simulink model "simsimulink"  (R2024a)
settings: Solver=ode8  StartTime=0.0  StopTime=10  FixedStep=0.000001  RelTol=1e-3
values from neighbouring files (symbols this model uses):
  am = 1/(Rlnom*C)    (= 53.1914893617)    [params.m]
  bm = 1    [params.m]
  C = 470e-6    (= 0.00047)    [params.m]
  E = 100    [params.m]
  k1 = 5000000    [params.m]
  k2 = 400000    [params.m]
  k3 = 700000    [params.m]
  kappa = 320    [params.m]
  L = 0.5e-3    (= 0.0005)    [params.m]
  omega = 100*pi    (= 314.159265359)    [params.m]
  Qas = bm    (= 1)    [params.m]
  R = 0.1    [params.m]
  Rlnom = 40    [params.m]
  Thetaas = 0    [params.m]
  vod = 200    [params.m]
  w = 100    [params.m]
libraries: spsIGBTDiodeLib x6, spsVoltageMeasurementLib x5, spsCurrentMeasurementLib x4, spsSeriesRLCBranchLib x4, spsACVoltageSourceLib x3, simulink x3, eeTransforms x2, spsControlledVoltageSourceLib x1, spsGroundLib x1, spsSVPWMGenerator2LevelLib x1, spsVariableResistorLib x1, spspowerguiLib x1
settings Model: Creator=rodol  LastModifiedBy=rodol

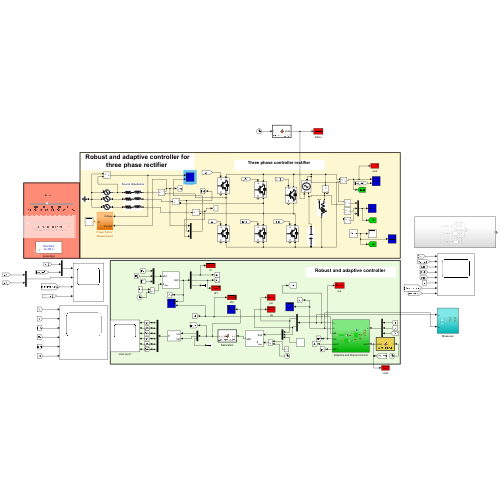
[thumbnail: Simulink's stored preview of the top-level diagram]
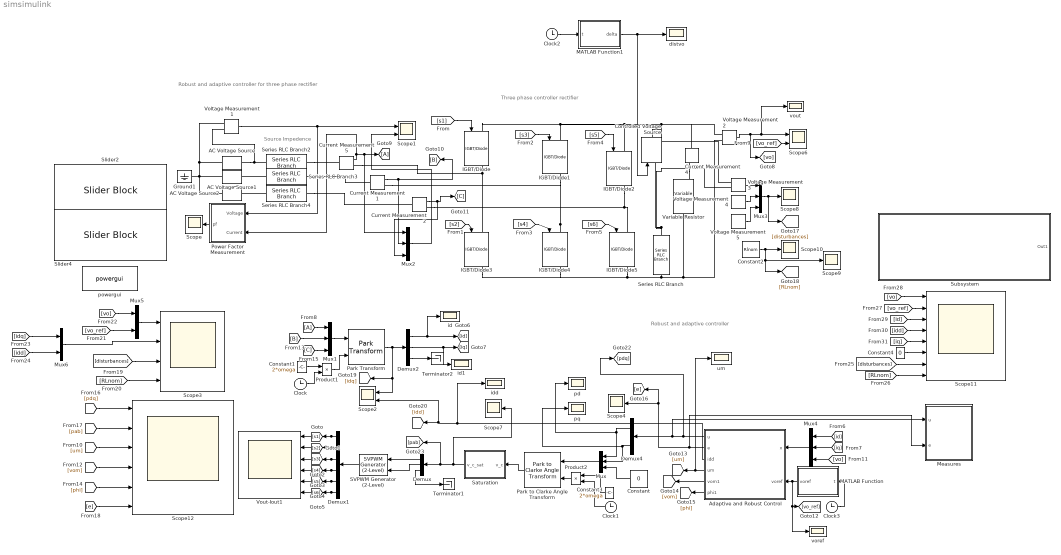
== system simsimulink ==
  note: Robust and adaptive controller
  note: Three phase controller rectifier
  note: Source Impedence
  note: Robust and adaptive controller for three phase rectifier
  " pq" : Scope
  AC Voltage Source : spsACVoltageSourceLib/AC Voltage Source  Amplitude=E  Phase=0  Frequency=w  SampleTime=0  Measurements=None  BusType=swing  Pref=10e3  Qref=0  Qmin=-inf  Qmax=+inf
  AC Voltage Source1 : spsACVoltageSourceLib/AC Voltage Source  Amplitude=E  Phase=240  Frequency=w  SampleTime=0  Measurements=None  BusType=swing  Pref=10e3  Qref=0  Qmin=-inf  Qmax=+inf
  AC Voltage Source2 : spsACVoltageSourceLib/AC Voltage Source  Amplitude=E  Phase=120  Frequency=w  SampleTime=0  Measurements=None  BusType=swing  Pref=10e3  Qref=0  Qmin=-inf  Qmax=+inf
  Adaptive and Robust Control : Subsystem
  Clock{,1..3} (4 alike) : Clock
  Constant : Constant  Value=0
  Constant1 : Constant  Value=2*omega
  Constant2 : Constant  Value=Rlnom
  Constant3 : Constant  Value=2*omega
  Constant4 : Constant  Value=0
  Controlled Voltage Source : spsControlledVoltageSourceLib/Controlled Voltage Source  Initialize=on  Source_Type=DC  Amplitude=0  Phase=0  Frequency=0  Measurements=None
  Current Measurement{1..2,4..5} (4 alike) : spsCurrentMeasurementLib/Current Measurement  PhasorSimulation=off  OutputType=Magnitude  PSBequivalent=0
  Demux : Demux  Outputs=3
  Demux1 : Demux  Outputs=6
  Demux2 : Demux  Outputs=3
  Demux4 : Demux  Outputs=2
  From8 : From
  Goto9 : Goto
  Ground1 : spsGroundLib/Ground  LConnTagsString=a
  IGBT/Diode{,1..5} (6 alike) : spsIGBTDiodeLib/IGBT//Diode  Ron=1e-3  Rs=1e5  Cs=inf  Measurements=on
  MATLAB Function : MATLAB Function  TreatAsAtomicUnit=on
  MATLAB Function1 : MATLAB Function  TreatAsAtomicUnit=on
  Measures : Subsystem
  Mux{,1..4} (5 alike) : Mux  Inputs=3
  Mux5 : Mux  Inputs=2
  Mux6 : Mux  Inputs=2
  Park Transform : eeTransforms/Park Transform  AxisAlignment=D-axis  PowerInvariant=off
  Park to Clarke Angle Transform : eeTransforms/Park to Clarke Angle Transform  AxisAlignment=D-axis
  Power Factor Measurement : Subsystem
  Product1 : Product
  Product2 : Product
  SVPWM Generator (2-Level) : spsSVPWMGenerator2LevelLib/SVPWM Generator (2-Level)  InputType=alpha-beta components  SwitchingPattern=Pattern #1  Fc=80000  ParUref=[0.8 -30 50]  Ts=0.000001
  Saturation : MATLAB Function  TreatAsAtomicUnit=on
  Scope{,4,7..10} (6 alike) : Scope
  Scope1 : Scope  NumInputPorts=2
  Scope11 : Scope  NumInputPorts=8
  Scope12 : Scope  NumInputPorts=6
  Scope2 : Scope  NumInputPorts=2
  Scope3 : Scope  NumInputPorts=4
  Scope6 : Scope  NumInputPorts=2
  Series RLC Branch : spsSeriesRLCBranchLib/Series RLC Branch  LConnTagsString=__new0  RConnTagsString=__new0  BranchType=C  Resistance=5  Inductance=1e-3  SetiL0=off  InitialCurrent=0  Capacitance=C  Setx0=off  InitialVoltage=0  Measurements=None
  Series RLC Branch2 : spsSeriesRLCBranchLib/Series RLC Branch  LConnTagsString=__new0  RConnTagsString=__new0  BranchType=RL  Resistance=R  Inductance=L  SetiL0=off  InitialCurrent=0  Capacitance=200e-6  Setx0=off  InitialVoltage=0  Measurements=Branch voltage and current
  Series RLC Branch3 : spsSeriesRLCBranchLib/Series RLC Branch  LConnTagsString=__new0  RConnTagsString=__new0  BranchType=RL  Resistance=R  Inductance=L  SetiL0=off  InitialCurrent=0  Capacitance=200e-6  Setx0=off  InitialVoltage=0  Measurements=Branch voltage and current
  Series RLC Branch4 : spsSeriesRLCBranchLib/Series RLC Branch  LConnTagsString=__new0  RConnTagsString=__new0  BranchType=RL  Resistance=R  Inductance=L  SetiL0=off  InitialCurrent=0  Capacitance=200e-6  Setx0=off  InitialVoltage=0  Measurements=Branch voltage and current
  Slider2 : SliderBlock  ScaleMin=25
  Slider4 : SliderBlock  ScaleMax=5
  Subsystem : Subsystem
  Terminator1 : Terminator
  Terminator2 : Terminator
  Variable Resistor : spsVariableResistorLib/Variable Resistor  Rabsmin=Rlnom
  Voltage Measurement{1..5} (5 alike) : spsVoltageMeasurementLib/Voltage Measurement  PhasorSimulation=off  OutputType=Magnitude  PSBequivalent=0
  Vout-Iout1 : Scope  NumInputPorts=6
  distvo : Scope
  id : Scope
  id1 : Scope
  idd : Scope
  pd : Scope
  powergui : spspowerguiLib/powergui  Priority=1  SimulationMode=Discrete  SampleTime=1e-6  frequency=60  Iterations=50  frequencyindice=0  Pbase=100e6  ErrMax=1e-4  UnitsV=kV  UnitsW=MW  buscounter=0  FunctionMessages=off  echomessages=off  EnableUseOfTLC=off  CurrentSourceSwitches=off  DisableSnubberDevices=off  DisableRonSwitches=off  DisableVfSwitches=off  DisplayEquations=off  AutomaticDiscreteSolvers=off  SolverType=Tustin/Backward Euler (TBE)  Interpol=off  ExternalGateDelay=off  methode=off  Ts=0  x0status=blocks  SPID=off  SwTol=0  HookPort=off  NonlinearTolerance=0  nMaxIteration=15  ContinueOnMaxIteration=off  RestoreLinks=warning  ResistiveCurrentMeasurement=off  Frange=[0:2:500]  Ylog=off  Xlog=on  ShowGrid=off  save=off  variable=ZData  structure=0  ZoomFFT=on  StartTime=0.0  cycles=1  DisplayStyle=1  fundamental=60  FreqAxis=off  MaxFrequency=1000  frequencyindicesteady=1  RmsSteady=1  display=off
  um : Scope
  voref : Scope
  vout : Scope
  wires:
  Demux2/2 -> id1/1, [iq]
  Clock1/1 -> Product2/2
  Park Transform/1 -> [idq], Scope2/1, Demux2/1
  Current Measurement5/1 -> Mux2/1, Goto9/1, Power Factor Measurement/2(Current)
  [s5] -> IGBT/Diode2/1
  [s4] -> IGBT/Diode4/1
  Demux1/5 -> Vout-Iout1/5, [s5]
  Product1/1 -> Park Transform/2
  Constant1/1 -> Product1/1
  Demux1/1 -> Vout-Iout1/1, [s1]
  [s2] -> IGBT/Diode3/1
  Clock/1 -> Product1/2
  Demux2/1 -> id/1, [id]
  [s1] -> IGBT/Diode/1
  Power Factor Measurement/1(pf) -> Scope/1
  Demux2/3 -> Terminator2/1
  [s6] -> IGBT/Diode5/1
  Mux1/1 -> Park Transform/1
  Constant3/1 -> Product2/1
  Product2/1 -> Park to Clarke Angle Transform/2
  Demux1/3 -> Vout-Iout1/3, [s3]
  Demux1/4 -> Vout-Iout1/4, [s4]
  Demux1/2 -> Vout-Iout1/2, [s2]
  Demux/3 -> Terminator1/1
  Constant/1 -> Mux/3
  Voltage Measurement1/1 -> Scope1/1, Power Factor Measurement/1(Voltage)
  Demux1/6 -> Vout-Iout1/6, [s6]
  [s3] -> IGBT/Diode1/1
  Demux4/1 -> pd/1, Mux/1
  Demux4/2 -> " pq"/1, Mux/2
  Voltage Measurement2/1 -> [vo], vout/1, Scope6/1
  Mux4/1 -> Adaptive and Robust Control/1(x)
  Clock3/1 -> MATLAB Function/1(t)
  MATLAB Function/1(voref) -> voref/1, [vo_ref], Adaptive and Robust Control/2(voref)
  [vo] -> Mux4/3
  [id] -> Mux4/1
  [iq] -> Mux4/2
  From8/1 -> Mux1/1
  Current Measurement1/1 -> Mux2/2, [B]
  [B] -> Mux1/2
  Current Measurement2/1 -> Mux2/3, [C]
  [C] -> Mux1/3
  [vo_ref] -> Scope6/2
  Mux2/1 -> Scope1/2
  Mux/1 -> Park to Clarke Angle Transform/1
  Adaptive and Robust Control/3(idd) -> idd/1, [idd], Scope2/2
  Voltage Measurement3/1 -> Mux3/1
  Voltage Measurement4/1 -> Mux3/2
  Voltage Measurement5/1 -> Mux3/3
  Mux3/1 -> [disturbances], Scope8/1
  Constant2/1 -> Scope9/1, [RLnom], Scope10/1
  Adaptive and Robust Control/4(um) -> um/1, [um]
  Adaptive and Robust Control/6(phi1) -> [phi]
  Adaptive and Robust Control/5(vom1) -> [vom]
  [um] -> Scope12/3
  [vom] -> Scope12/4
  [phi] -> Scope12/5
  [pdq] -> Scope12/1
  [e] -> Scope12/6
  [vo] -> Mux5/1
  [vo_ref] -> Mux5/2
  [idq] -> Mux6/1
  [idd] -> Mux6/2
  Mux5/1 -> Scope3/1
  Mux6/1 -> Scope3/2
  [disturbances] -> Scope3/3
  [RLnom] -> Scope3/4
  [vo] -> Scope11/1
  [vo_ref] -> Scope11/2
  [id] -> Scope11/3
  [iq] -> Scope11/5
  [idd] -> Scope11/4
  Constant4/1 -> Scope11/6
  [disturbances] -> Scope11/7
  [RLnom] -> Scope11/8
  [pab] -> Scope12/2
  Clock2/1 -> MATLAB Function1/1(t)
  MATLAB Function1/1(delta) -> distvo/1, Controlled Voltage Source/1
  Adaptive and Robust Control/2(e) -> Measures/2(e), [e], Scope4/1
  Adaptive and Robust Control/1(u) -> [pdq], Measures/1(u), Demux4/1
  Demux/1 -> SVPWM Generator (2-Level)/1
  Demux/2 -> SVPWM Generator (2-Level)/2
  Park to Clarke Angle Transform/1 -> Saturation/1(v_c)
  SVPWM Generator (2-Level)/1 -> Demux1/1
  Saturation/1(v_c_sat) -> Scope7/1, [pab], Demux/1
  connections:
  IGBT/Diode1/LConn1 -- IGBT/Diode/LConn1 -- Voltage Measurement3/LConn1 -- Controlled Voltage Source/RConn1 -- Current Measurement4/LConn1 -- Voltage Measurement2/LConn1 -- IGBT/Diode2/LConn1
  IGBT/Diode2/RConn1 -- IGBT/Diode5/LConn1 -- Current Measurement2/RConn1
  Series RLC Branch3/RConn1 -- Current Measurement1/LConn1
  Series RLC Branch2/RConn1 -- Current Measurement5/LConn1
  Series RLC Branch4/RConn1 -- Current Measurement2/LConn1
  AC Voltage Source/RConn1 -- Voltage Measurement1/LConn1 -- AC Voltage Source2/RConn1 -- AC Voltage Source1/RConn1 -- Ground1/LConn1
  IGBT/Diode4/LConn1 -- IGBT/Diode1/RConn1 -- Current Measurement1/RConn1
  Current Measurement5/RConn1 -- IGBT/Diode/RConn1 -- IGBT/Diode3/LConn1
  Series RLC Branch3/LConn1 -- AC Voltage Source1/LConn1
  Voltage Measurement2/LConn2 -- IGBT/Diode4/RConn1 -- IGBT/Diode3/RConn1 -- IGBT/Diode5/RConn1 -- Series RLC Branch/RConn1 -- Variable Resistor/RConn1
  Series RLC Branch4/LConn1 -- AC Voltage Source2/LConn1
  AC Voltage Source/LConn1 -- Voltage Measurement1/LConn2 -- Series RLC Branch2/LConn1
  Current Measurement4/RConn1 -- Variable Resistor/LConn1
  Series RLC Branch/LConn1 -- Voltage Measurement3/LConn2 -- Controlled Voltage Source/LConn1

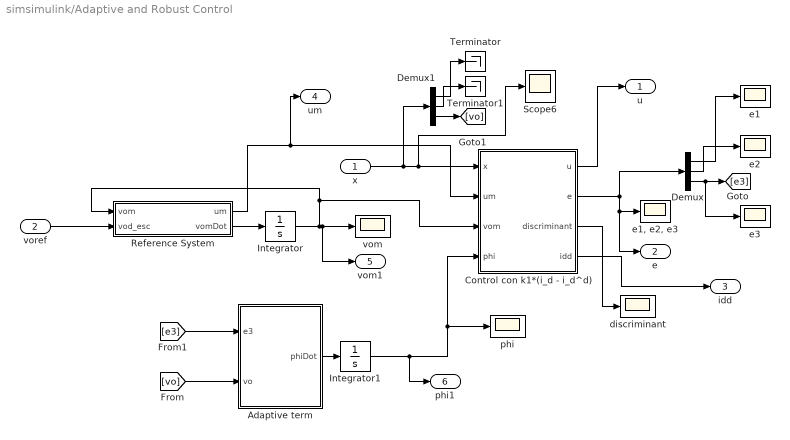
== system simsimulink/Adaptive and Robust Control ==
  x : Inport
  voref : Inport  Port=2
  " e1" : Scope
  " e2" : Scope
  " e3" : Scope
  Adaptive term : MATLAB Function  TreatAsAtomicUnit=on
  Control con k1*(i_d - i_d^d) : MATLAB Function  TreatAsAtomicUnit=on
  Demux : Demux  Outputs=3
  Demux1 : Demux  Outputs=3
  Integrator : Integrator
  Integrator1 : Integrator
  Reference System : MATLAB Function  TreatAsAtomicUnit=on
  Scope6 : Scope
  Terminator : Terminator
  Terminator1 : Terminator
  discriminant : Scope
  "e1, e2, e3" : Scope
  phi : Scope
  vom : Scope
  u : Outport
  e : Outport  Port=2
  idd : Outport  Port=3
  um : Outport  Port=4
  vom1 : Outport  Port=5
  phi1 : Outport  Port=6
  wires:
  x/1 -> Demux1/1, Scope6/1, Control con k1*(i_d - i_d^d)/1(x)
  Control con k1*(i_d - i_d^d)/3(discriminant) -> discriminant/1
  Control con k1*(i_d - i_d^d)/2(e) -> e/1, "e1, e2, e3"/1, Demux/1
  Control con k1*(i_d - i_d^d)/1(u) -> u/1
  Reference System/2(vomDot) -> Integrator/1
  Integrator/1 -> vom1/1, vom/1, Reference System/1(vom), Control con k1*(i_d - i_d^d)/3(vom)
  Adaptive term/1(phiDot) -> Integrator1/1
  Reference System/1(um) -> um/1, Control con k1*(i_d - i_d^d)/2(um)
  Integrator1/1 -> phi1/1, phi/1, Control con k1*(i_d - i_d^d)/4(phi)
  Demux/3 -> " e3"/1, [e3]
  Demux1/3 -> [vo]
  [e3] -> Adaptive term/1(e3)
  [vo] -> Adaptive term/2(vo)
  Demux1/1 -> Terminator/1
  Demux1/2 -> Terminator1/1
  voref/1 -> Reference System/2(vod_esc)
  Demux/1 -> " e1"/1
  Demux/2 -> " e2"/1
  Control con k1*(i_d - i_d^d)/4(idd) -> idd/1

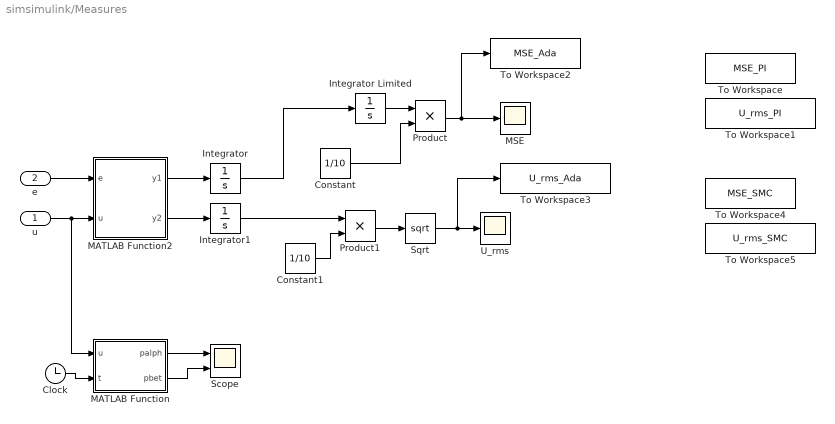
== system simsimulink/Measures ==
  u : Inport
  e : Inport  Port=2
  Clock : Clock
  Constant : Constant  Value=1/10
  Constant1 : Constant  Value=1/10
  Integrator : Integrator
  Integrator Limited : Integrator  UpperSaturationLimit=1  LowerSaturationLimit=0
  Integrator1 : Integrator
  MATLAB Function : MATLAB Function  TreatAsAtomicUnit=on
  MATLAB Function2 : MATLAB Function  TreatAsAtomicUnit=on
  MSE : Scope
  Product : Product
  Product1 : Product
  Scope : Scope  NumInputPorts=2
  Sqrt : Sqrt
  To Workspace : ToWorkspace  VariableName=MSE_PI  SaveFormat=Timeseries  SampleTime=-1
  To Workspace1 : ToWorkspace  VariableName=U_rms_PI  SaveFormat=Timeseries  SampleTime=-1
  To Workspace2 : ToWorkspace  VariableName=MSE_Ada  SaveFormat=Timeseries  SampleTime=-1
  To Workspace3 : ToWorkspace  VariableName=U_rms_Ada  SaveFormat=Timeseries  SampleTime=-1
  To Workspace4 : ToWorkspace  VariableName=MSE_SMC  SaveFormat=Timeseries  SampleTime=-1
  To Workspace5 : ToWorkspace  VariableName=U_rms_SMC  SaveFormat=Timeseries  SampleTime=-1
  U_rms : Scope
  wires:
  Integrator Limited/1 -> Product/1
  Constant/1 -> Product/2
  Product/1 -> To Workspace2/1, MSE/1
  Sqrt/1 -> To Workspace3/1, U_rms/1
  MATLAB Function2/2(y2) -> Integrator1/1
  Constant1/1 -> Product1/2
  Product1/1 -> Sqrt/1
  u/1 -> MATLAB Function/1(u), MATLAB Function2/2(u)
  e/1 -> MATLAB Function2/1(e)
  MATLAB Function2/1(y1) -> Integrator/1
  Integrator/1 -> Integrator Limited/1
  Integrator1/1 -> Product1/1
  Clock/1 -> MATLAB Function/2(t)
  MATLAB Function/1(palph) -> Scope/1
  MATLAB Function/2(pbet) -> Scope/2

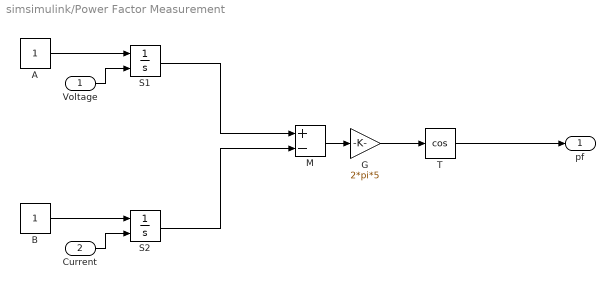
== system simsimulink/Power Factor Measurement ==
  Voltage : Inport
  Current : Inport  Port=2
  A : Constant
  B : Constant
  G : Gain  Gain=2*pi*5
  M : Sum  Inputs=+-
  S1 : Integrator  ExternalReset=falling
  S2 : Integrator  ExternalReset=falling
  T : Trigonometry  Operator=cos
  pf : Outport
  wires:
  A/1 -> S1/1
  B/1 -> S2/1
  S1/1 -> M/1
  S2/1 -> M/2
  Voltage/1 -> S1/2
  Current/1 -> S2/2
  M/1 -> G/1
  G/1 -> T/1
  T/1 -> pf/1

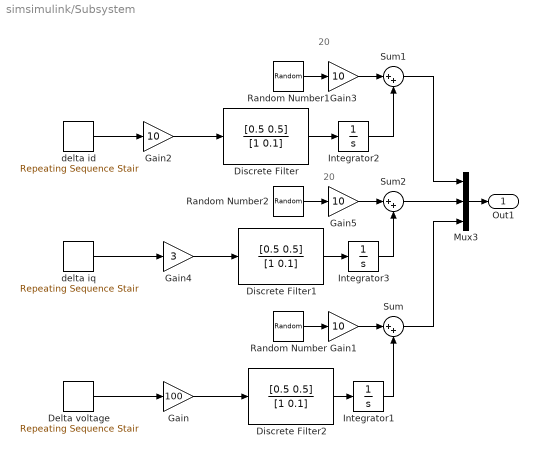
== system simsimulink/Subsystem ==
  note: 20
  note: 20
  Delta voltage : simulink/Sources/Repeating Sequence Stair  OutValues=[0 0 1 1 -1 2 -5 -5 -4 1 5 6 7 4].'  tsamp=0.5  OutMin=[]  OutMax=[]  OutDataTypeStr=double  OutputDataTypeScalingMode=double  OutDataType=fixdt(0,8)  ConRadixGroup=Best Precision: Vector-wise  OutScaling=2^-12
  Discrete Filter : DiscreteFilter  Numerator=[0.5 0.5]  Denominator=[1 0.1]  InputProcessing=Columns as channels (frame based)  FilterStructure=Direct form II transposed  a0EqualsOne=on
  Discrete Filter1 : DiscreteFilter  Numerator=[0.5 0.5]  Denominator=[1 0.1]  InputProcessing=Columns as channels (frame based)  FilterStructure=Direct form II transposed  a0EqualsOne=on
  Discrete Filter2 : DiscreteFilter  Numerator=[0.5 0.5]  Denominator=[1 0.1]  InputProcessing=Columns as channels (frame based)  FilterStructure=Direct form II transposed  a0EqualsOne=on
  Gain : Gain  Gain=100
  Gain{1..3,5} (4 alike) : Gain  Gain=10
  Gain4 : Gain  Gain=3
  Integrator1 : Integrator
  Integrator2 : Integrator
  Integrator3 : Integrator
  Mux3 : Mux  Inputs=3
  Random Number : RandomNumber  SampleTime=0.01
  Random Number1 : RandomNumber  SampleTime=0.01
  Random Number2 : RandomNumber  SampleTime=0.01
  Sum : Sum  Inputs=|++
  Sum1 : Sum  Inputs=|++
  Sum2 : Sum  Inputs=|++
  delta id : simulink/Sources/Repeating Sequence Stair  OutValues=[-3 -4 -7 -7 -1 2 5 5 4 6 3 2 1 0].'  tsamp=0.5  OutMin=[]  OutMax=[]  OutDataTypeStr=double  OutputDataTypeScalingMode=double  OutDataType=fixdt(0,8)  ConRadixGroup=Best Precision: Vector-wise  OutScaling=2^-12
  delta iq : simulink/Sources/Repeating Sequence Stair  OutValues=[1 2 3 4 4 4 5 5 4 4 3 3 3 3].'  tsamp=0.5  OutMin=[]  OutMax=[]  OutDataTypeStr=double  OutputDataTypeScalingMode=double  OutDataType=fixdt(0,8)  ConRadixGroup=Best Precision: Vector-wise  OutScaling=2^-12
  Out1 : Outport
  wires:
  Random Number/1 -> Gain1/1
  Random Number1/1 -> Gain3/1
  Gain/1 -> Discrete Filter2/1
  Gain5/1 -> Sum2/1
  Gain1/1 -> Sum/1
  Integrator3/1 -> Sum2/2
  Sum/1 -> Mux3/3
  Sum1/1 -> Mux3/1
  Discrete Filter1/1 -> Integrator3/1
  Random Number2/1 -> Gain5/1
  Sum2/1 -> Mux3/2
  Discrete Filter2/1 -> Integrator1/1
  Integrator2/1 -> Sum1/2
  Delta voltage/1 -> Gain/1
  delta iq/1 -> Gain4/1
  delta id/1 -> Gain2/1
  Gain3/1 -> Sum1/1
  Discrete Filter/1 -> Integrator2/1
  Integrator1/1 -> Sum/2
  Gain2/1 -> Discrete Filter/1
  Gain4/1 -> Discrete Filter1/1
  Mux3/1 -> Out1/1

== matlab function simsimulink/Saturation ==
  data: v_c input; v_c_sat output
function v_c_sat = saturateVector(v_c)
%#codegen

% Separar componentes del vector
p_alpha = v_c(1);
p_beta = v_c(2);

% Calcular la magnitud
v_mag = sqrt(p_alpha^2 + p_beta^2);

% Máxima magnitud permitida
V_max = 0.866;

% Escalado si excede el límite
if v_mag <= V_max
    v_c_sat = v_c;
else
    scale = V_max / v_mag;
    v_c_sat = v_c * scale;
end

== matlab function simsimulink/Adaptive and Robust Control/Reference System ==
  data: um output; vom input; vomDot output; am parameter; bm parameter; kappa parameter; vod_esc input
function [um, vomDot] = ref(vom, am, bm, kappa, vod_esc)

% Control
um = (1/bm)*( am*vom - kappa*(vom - vod_esc) );

% System
vomDot = - am*vom + bm*um ;

== matlab function simsimulink/MATLAB Function1 ==
  settings: updateMethod=DISCRETE
  data: t input; delta output
function delta = disturbance_signal(t)
% Disturbance and load variation signal approximation

% Componente suave (función senoidal con pendiente)
delta_base = 30*sin(0.7*t) + 5*t -20;

% Componente de ruido o pequeñas variaciones escalonadas:
% (simulando pequeños saltos pseudo-aleatorios)
rng(1); % Para reproducibilidad
persistent steps times
if isempty(steps)
    times = 0:0.09:10;
    steps = 0.1*(randn(size(times))); % valores aleatorios pequeños
end

% Interpolación para el valor de la señal escalonada en el tiempo t
noise_val = interp1(times, steps, t, 'previous', 0);

% Combinación final
delta = delta_base + noise_val;

end

== matlab function simsimulink/Adaptive and Robust Control/Control con k1*(i_d - i_d^d) ==
  data: x input; um input; vom input; phi input; u output; k1 parameter; k2 parameter; k3 parameter; vod parameter; R parameter; L parameter; C parameter; Rlnom parameter; omega parameter; E parameter; e output; discriminant output; Thetaas parameter; Qas parameter; idd output
function [u, e, discriminant,idd] = ctrl(x, um, vom, phi, k1, k2, k3, vod, R, L, C, Rlnom, omega, E, Thetaas, Qas)

id = x(1,1);
iq = x(2,1); 
vo = x(3,1);

% Errors e2, e3
e2 = iq;        e3 = vo - vom;
Theta = phi + Thetaas;

% Controls [Adaptive terms]
pq = ( (2*L)/(e3 + vom) )*( - (R/L)*iq - omega*id + k2*e2 ) ; % k2*e2 , k2*sqrt(abs(e2))*sign(e2)
v2 = Theta*vo + Qas*um  - (3/(4*C))*(iq*pq) - k3*e3 ;  % k3*e3 , k3*sqrt(abs(e3))*sign(e3)
%
%pq = ( 2*L/vo )*( - (R/L)*iq - omega*id + k2*sqrt(abs(e2))*sign(e2) ) ; % k2*e2 , k2*sqrt(abs(e2))*sign(e2)
%v2 = - (3/(4*C))*(iq*pq) + (1/(Rl*C))*vo - k3*sqrt(abs(e3))*sign(e3) ;  % k3*e3 , k3*sqrt(abs(e3))*sign(e3)

% Combinando las sigs. eqs (23) [version no adaptiva]
% pd = ((2*L)/(vo)) * ( - (R/L)*id + omega*iq + (E/L) + k1*(id - idd) ) ;
% idd = (4*C*v2)/(3*pd) ; 
% obtenemos:

a = k1;
b = (R/L) * id - omega * iq - (E/L) - k1 * id;
c = (2 * C * v2 * vo) / (3 * L);
discriminant = b^2 - 4 * a * c; %no debe ser cero

idd = ( -b + sqrt(b^2 - 4 * a * c) ) / (2 * a); %id deseada dinamica

pd = (4 * C * v2) / (3 * idd); %sale de (23)------------------> CONTROL REAL

% Error e1
e1 = id - idd;


% Salidas
u = [pd;
     pq];

e = [e1;
     e2;
     e3];

== matlab function simsimulink/Adaptive and Robust Control/Adaptive term ==
  data: e3 input; phiDot output; vo input; lambda parameter
function phiDot = fcn(e3, vo, lambda)


phiDot = - lambda*e3*vo;

== matlab function simsimulink/MATLAB Function ==
  data: t input; voref output; vod parameter
function voref = step_signal(t, vod)
% Generates a step signal increasing from 160 to 220 in steps of 20
% over a simulation time of 0 to 10 seconds.

    % Define step times and corresponding values
    %step_times = [0, 3.3, 6.6, 10]; % Change points
    %step_values = [vod-40, vod-20, vod, vod]; % Corresponding values
    step_times = [0, 2, 4, 6, 8]; % Change points
    %step_values = [vod-40, vod-20, vod, vod+20, vod+40]; % Corresponding values
    step_values = [vod, vod+20, vod+40, vod+80, vod+40]; % Corresponding values
    
    % Initialize output
    voref = step_values(1);
    
    % Apply step changes
    for i = 2:length(step_times)
        if t >= step_times(i)
            voref = step_values(i);
        end
    end
end

== matlab function simsimulink/Measures/MATLAB Function ==
  data: u input; palph output; t input; pbet output; omega parameter
function [palph, pbet] = fcn(u, t, omega)

pd = u(1,1);
pq = u(2,1);

theta = omega*t;

A = [ cos(theta), sin(theta);
     -sin(theta), cos(theta)];


a = A*[pd;pq];

palph = a(1,1);
pbet = a(2,1);

== matlab function simsimulink/Measures/MATLAB Function2 ==
  data: e input; y1 output; u input; y2 output
function [y1, y2] = fcn(e, u)

e1 = e(1,1);
e2 = e(2,1);
e3 = e(3,1);

pd = u(1,1);
pq = u(2,1);

y1 = e2^2 + e3^2;
y2 = pd^2 + pq^2;
